simulink model "Stanley_Regler"  (R2019b)
settings: Solver=VariableStepAuto  StartTime=0.0  StopTime=10.0  RelTol=1e-3
libraries: drivingvehiclecontroller x2

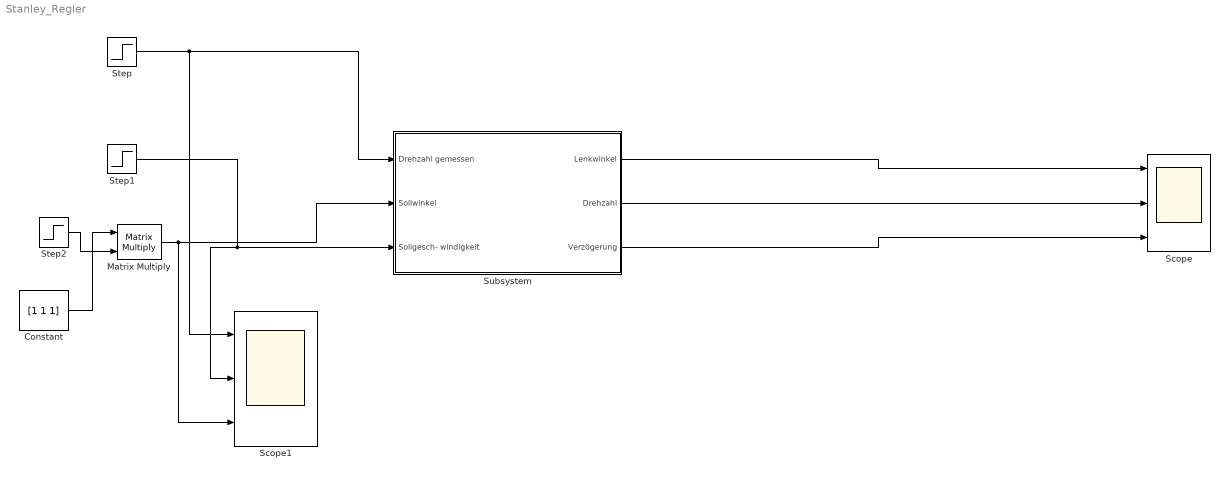
== system Stanley_Regler ==
  Constant : Constant  Value=[1 1 1]
  Matrix Multiply : Product  Multiplication=Matrix(*)
  Scope : Scope  NumInputPorts=3
  Scope1 : Scope  NumInputPorts=3
  Step : Step  After=100  SampleTime=0
  Step1 : Step  After=10  SampleTime=0
  Step2 : Step  After=18  SampleTime=0
  Subsystem : Subsystem
  wires:
  Step/1 -> Scope1/1, Subsystem/1(Drehzahl gemessen)
  Step1/1 -> Scope1/2, Subsystem/3(Sollgesch- windigkeit)
  Subsystem/1(Lenkwinkel) -> Scope/1
  Subsystem/2(Drehzahl) -> Scope/2
  Subsystem/3(Verzögerung) -> Scope/3
  Matrix Multiply/1 -> Scope1/3, Subsystem/2(Sollwinkel)
  Constant/1 -> Matrix Multiply/1
  Step2/1 -> Matrix Multiply/2

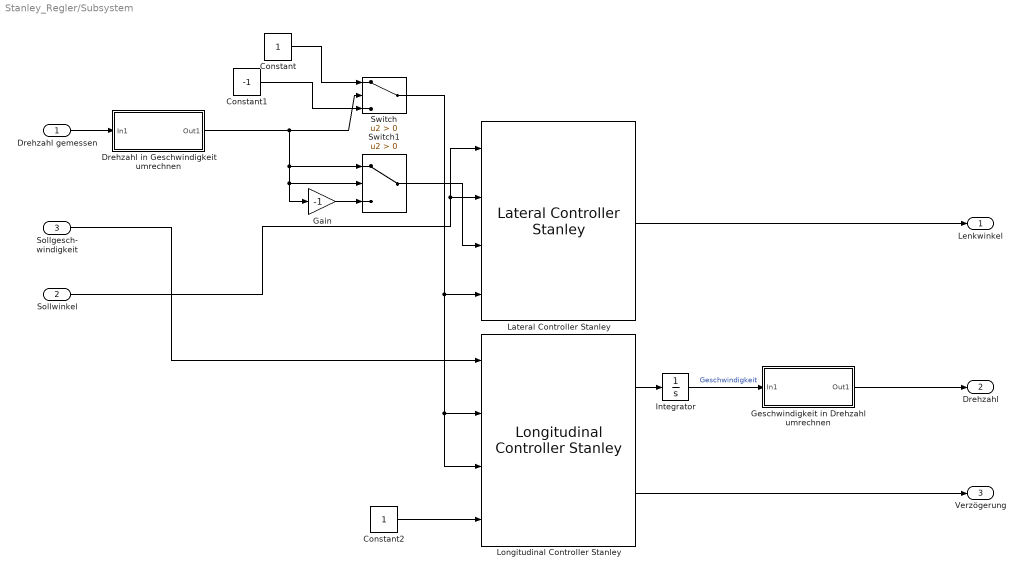
== system Stanley_Regler/Subsystem ==
  Drehzahl gemessen : Inport
  Sollwinkel : Inport  Port=2
  Sollgesch- windigkeit : Inport  Port=3
  Constant : Constant
  Constant1 : Constant  Value=-1
  Constant2 : Constant
  Drehzahl in Geschwindigkeit umrechnen : Subsystem
  Gain : Gain  Gain=-1
  "Geschwindigkeit in Drehzahl umrechnen " : Subsystem
  Integrator : Integrator
  Lateral Controller Stanley : drivingvehiclecontroller/Lateral Controller Stanley  ModelType=Kinematic bicycle model  PositionGainF=2.5  PositionGainR=2.5  YawRateGain=0.2  DelayGain=0.2  VehicleMass=1575  Lf=1.2  Lr=1.6  TireStiffness=19000  Wheelbase=2.8  MaxSteeringAngle=20
  Longitudinal Controller Stanley : drivingvehiclecontroller/Longitudinal Controller Stanley  Kp=2.5  Ki=1  SampleTime=0.05  MaxAcceleration=3  MaxDeceleration=1
  Switch : Switch  Criteria=u2 > Threshold
  Switch1 : Switch  Criteria=u2 > Threshold
  Lenkwinkel : Outport
  Drehzahl : Outport  Port=2
  Verzögerung : Outport  Port=3
  wires:
  Sollgesch- windigkeit/1 -> Longitudinal Controller Stanley/1
  Switch1/1 -> Lateral Controller Stanley/3
  Drehzahl in Geschwindigkeit umrechnen/1(Out1) -> Switch/2, Switch1/1, Gain/1, Switch1/2
  Drehzahl gemessen/1 -> Drehzahl in Geschwindigkeit umrechnen/1(In1)
  Constant/1 -> Switch/1
  Sollwinkel/1 -> Lateral Controller Stanley/1, Lateral Controller Stanley/2
  "Geschwindigkeit in Drehzahl umrechnen "/1(Out1) -> Drehzahl/1
  Switch/1 -> Longitudinal Controller Stanley/2, Longitudinal Controller Stanley/3, Lateral Controller Stanley/4
  Gain/1 -> Switch1/3
  Lateral Controller Stanley/1 -> Lenkwinkel/1
  Constant1/1 -> Switch/3
  Integrator/1 -> "Geschwindigkeit in Drehzahl umrechnen "/1(In1)  "Geschwindigkeit"
  Constant2/1 -> Longitudinal Controller Stanley/4
  Longitudinal Controller Stanley/1 -> Integrator/1
  Longitudinal Controller Stanley/2 -> Verzögerung/1

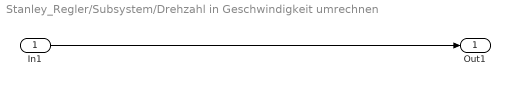
== system Stanley_Regler/Subsystem/Drehzahl in Geschwindigkeit umrechnen ==
  In1 : Inport
  Out1 : Outport
  wires:
  In1/1 -> Out1/1

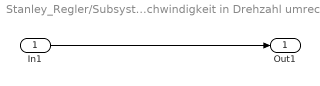
== system Stanley_Regler/Subsystem/Geschwindigkeit in Drehzahl umrechnen  ==
  In1 : Inport
  Out1 : Outport
  wires:
  In1/1 -> Out1/1
